simulink model "lazo_cerrado_cir"  (Simulink 7.6)
settings: Solver=VariableStepDiscrete  StartTime=0.0  StopTime=10.0  FixedStep=1e-3  MaxStep=1e-3  RelTol=1e0  AbsTol=1e1
values from neighbouring files (symbols this model uses):
  K = evalin('base','K')    [lazo_cerrado.m]    (also in linealizacion_dis.m = uquad_dlqr(Aext,Bext,Q,R); sim_lazo_cerrado.m = linealizacion_dis(modo,setpoint,0))
  setpoint = [evalin('base','vs') evalin('base','thetaps')]    [lazo_cerrado.m]    (also in programa_de_vuelo.m = [v(k,:) 0]; sim_lazo_cerrado.m = [ G(1) G(2) G(3) G(4) G(5) G(6) G(7) G(8)])
  thetap = evalin('base','thetap')    [linealizacion.m]
  ti = evalin('base','ti')    [lazo_cerrado.m]    (also in programa_de_vuelo.m = 0.1)
  Ts = evalin('base','Ts')    [linealizacion.m]    (also in linealizacion_dis.m)
undefined symbols (not defined in the file or in its folder): ang_amp, ang_frec, ang_offset, DiscIntNeverNeededParam, g, hor_amp, hor_frec, hor_offset, Ixx, Iyy, Izz, Izzm, L, M, phi0, psi0, theta0, vq10, vq20, vq30, vq_amp, vq_frec, vq_offset, wq10, wq20, wq30, wq_amp, wq_frec, wq_offset, x0, xc, y0, yaw_amp, yaw_frec, yaw_offset, yc, z0, z_amp, z_frec, z_offset, zc
libraries: commnoisgen2 x12, aerolibutil x3, simulink x1
settings Model: Creator=pater  LastModifiedBy=pater
settings SolverCC: InitialStep=0.01  MaxOrder=2  MaxConsecutiveMinStep=100  SolverJacobianMethodControl=FullPerturbation  SolverResetMethod=Robust
settings DataIOCC: SaveState=on
settings DebuggingCC: SignalInfNanChecking=error  MergeDetectMultiDrivingBlocksExec=warning

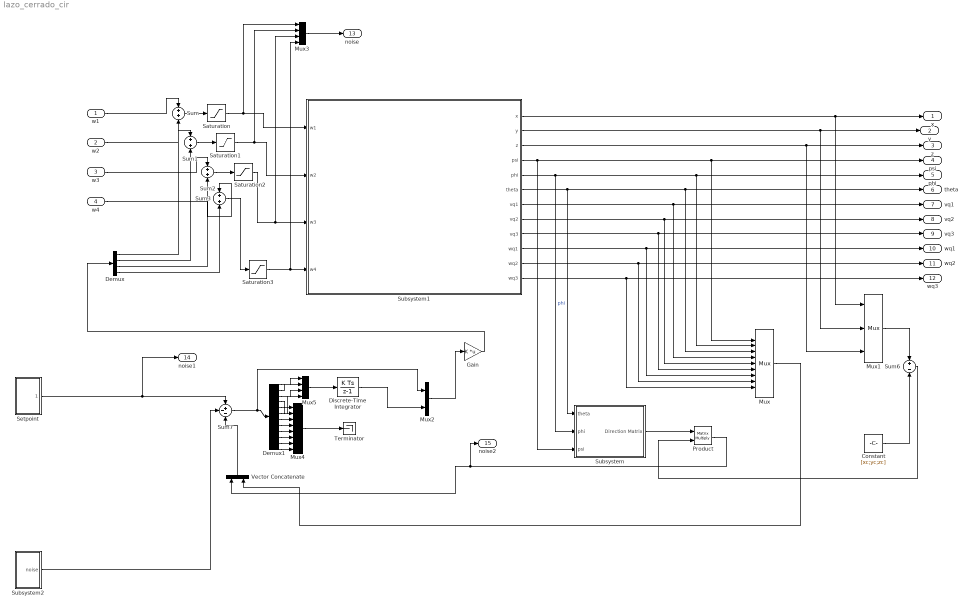
== system lazo_cerrado_cir ==
  w1 : Inport
  w2 : Inport  Port=2
  w3 : Inport  Port=3
  w4 : Inport  Port=4
  Constant : Constant  Value=[xc;yc;zc]
  Demux : Demux
  Demux1 : Demux  Outputs=12
  Discrete-Time Integrator : DiscreteIntegrator  SampleTime=Ts  UpperSaturationLimit=15  LowerSaturationLimit=-15  ICPrevOutput=DiscIntNeverNeededParam  ICPrevScaledInput=DiscIntNeverNeededParam
  Gain : Gain  Gain=K  Multiplication=Matrix(K*u) (u vector)
  Mux : Mux  Inputs=9
  Mux1 : Mux  Inputs=3
  Mux2 : Mux  Inputs=2
  Mux3 : Mux
  Mux4 : Mux  Inputs=8
  Mux5 : Mux
  Product : Product  Multiplication=Matrix(*)  RndMeth=Zero
  Saturation{,1..3} (4 alike) : Saturate  UpperLimit=387  LowerLimit=109
  Setpoint : Subsystem
  Subsystem : Subsystem
  Subsystem1 : Subsystem
  Subsystem2 : Subsystem
  Sum : Sum  OutMin=109.0  OutMax=387.0
  Sum1 : Sum  OutMin=109  OutMax=387
  Sum2 : Sum  OutMin=109  OutMax=387
  Sum3 : Sum  OutMin=109  OutMax=387
  Sum6 : Sum  Inputs=+-
  Sum7 : Sum  Inputs=+--
  Terminator : Terminator
  Vector Concatenate : Concatenate  Mode=Vector
  x : Outport
  y : Outport  Port=2
  z : Outport  Port=3  SampleTime=0.1
  psi : Outport  Port=4
  phi : Outport  Port=5
  theta : Outport  Port=6
  vq1 : Outport  Port=7
  vq2 : Outport  Port=8
  vq3 : Outport  Port=9
  wq1 : Outport  Port=10
  wq2 : Outport  Port=11
  wq3 : Outport  Port=12
  noise : Outport  Port=13
  noise1 : Outport  Port=14
  noise2 : Outport  Port=15
  wires:
  Subsystem1/1(x) -> x/1, Mux1/1
  Subsystem1/2(y) -> y/1, Mux1/2
  Subsystem1/3(z) -> z/1, Mux1/3
  Subsystem1/4(psi) -> psi/1, Mux/1, Subsystem/3(psi)
  Subsystem1/5(phi) -> Mux/2, phi/1, Subsystem/2(phi)  "phi"
  Subsystem1/6(theta) -> theta/1, Mux/3, Subsystem/1(theta)
  Subsystem1/7(vq1) -> vq1/1, Mux/4
  Subsystem1/8(vq2) -> vq2/1, Mux/5
  Subsystem1/9(vq3) -> vq3/1, Mux/6
  Subsystem1/10(wq1) -> wq1/1, Mux/7
  Subsystem1/11(wq2) -> wq2/1, Mux/8
  Subsystem1/12(wq3) -> wq3/1, Mux/9
  Mux/1 -> Vector Concatenate/2
  Mux1/1 -> Sum6/1
  Constant/1 -> Sum6/2
  Sum6/1 -> Product/2
  Subsystem/1(Direction Matrix) -> Product/1
  Demux/4 -> Sum3/2
  Demux/3 -> Sum2/2
  Demux/2 -> Sum1/2
  Demux/1 -> Sum/2
  w1/1 -> Sum/1
  w2/1 -> Sum1/1
  w3/1 -> Sum2/1
  w4/1 -> Sum3/1
  Sum3/1 -> Saturation3/1
  Sum2/1 -> Saturation2/1
  Sum1/1 -> Saturation1/1
  Sum/1 -> Saturation/1
  Saturation/1 -> Subsystem1/1(w1), Mux3/1
  Saturation1/1 -> Mux3/2, Subsystem1/2(w2)
  Saturation2/1 -> Subsystem1/3(w3), Mux3/3
  Saturation3/1 -> Subsystem1/4(w4), Mux3/4
  Gain/1 -> Demux/1
  Subsystem2/1(noise) -> Sum7/2
  Product/1 -> Vector Concatenate/1, noise2/1
  Sum7/1 -> Demux1/1, Mux2/1
  Mux4/1 -> Terminator/1
  Demux1/12 -> Mux4/8
  Demux1/11 -> Mux4/7
  Demux1/10 -> Mux4/6
  Demux1/9 -> Mux4/5
  Demux1/8 -> Mux4/4
  Demux1/7 -> Mux4/3
  Demux1/5 -> Mux4/2
  Demux1/4 -> Mux4/1
  Demux1/2 -> Mux5/2
  Demux1/1 -> Mux5/1
  Mux5/1 -> Discrete-Time Integrator/1
  Vector Concatenate/1 -> Sum7/3
  Setpoint/1(Setpoint) -> Sum7/1, noise1/1
  Mux3/1 -> noise/1
  Mux2/1 -> Gain/1
  Discrete-Time Integrator/1 -> Mux2/2
  Demux1/6 -> Mux5/4
  Demux1/3 -> Mux5/3

== system lazo_cerrado_cir/Setpoint ==
  Digital Clock : DigitalClock  SampleTime=Ts
  Product : Product  RndMeth=Zero
  Roll y Pitch : Constant  Value=[setpoint(4);setpoint(5)]
  Sum : Sum  Inputs=|++
  Sum1 : Sum  Inputs=|+-
  Vector Concatenate : Concatenate  NumInputs=4  Mode=Vector
  Vel y vel angular : Constant  Value=setpoint(6:11)
  Velocidad angular : Constant  Value=thetap
  angulo inicial : Constant  Value=theta0
  ti : Constant  Value=ti
  xq,yq,zq : Constant  Value=[setpoint(3);setpoint(2);setpoint(1)]
  Setpoint : Outport
  wires:
  Velocidad angular/1 -> Product/2
  Vector Concatenate/1 -> Setpoint/1
  angulo inicial/1 -> Sum/2
  ti/1 -> Sum1/2
  Digital Clock/1 -> Sum1/1
  Sum1/1 -> Product/1
  Product/1 -> Sum/1
  Vel y vel angular/1 -> Vector Concatenate/4
  Sum/1 -> Vector Concatenate/3
  Roll y Pitch/1 -> Vector Concatenate/2
  xq,yq,zq/1 -> Vector Concatenate/1

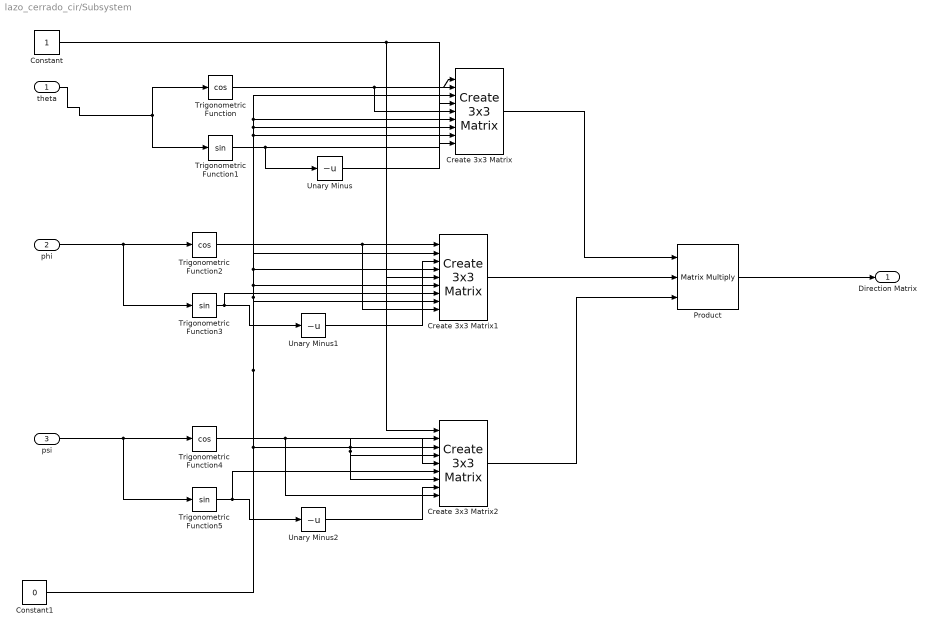
== system lazo_cerrado_cir/Subsystem ==
  theta : Inport
  phi : Inport  Port=2
  psi : Inport  Port=3
  Constant : Constant
  Constant1 : Constant  Value=0
  Create 3x3 Matrix : aerolibutil/Create 3x3 Matrix  SystemSampleTime=-1
  Create 3x3 Matrix1 : aerolibutil/Create 3x3 Matrix  SystemSampleTime=-1
  Create 3x3 Matrix2 : aerolibutil/Create 3x3 Matrix  SystemSampleTime=-1
  Product : Product  Inputs=3  Multiplication=Matrix(*)  RndMeth=Zero
  Trigonometric Function : Trigonometry  Operator=cos
  Trigonometric Function1 : Trigonometry
  Trigonometric Function2 : Trigonometry  Operator=cos
  Trigonometric Function3 : Trigonometry
  Trigonometric Function4 : Trigonometry  Operator=cos
  Trigonometric Function5 : Trigonometry
  Unary Minus : UnaryMinus
  Unary Minus1 : UnaryMinus
  Unary Minus2 : UnaryMinus
  Direction Matrix : Outport
  wires:
  Constant1/1 -> Create 3x3 Matrix/3, Create 3x3 Matrix/6, Create 3x3 Matrix/7, Create 3x3 Matrix/8, Create 3x3 Matrix1/2, Create 3x3 Matrix1/4, Create 3x3 Matrix1/6, Create 3x3 Matrix1/8, Create 3x3 Matrix2/3, Create 3x3 Matrix2/2, Create 3x3 Matrix2/7, Create 3x3 Matrix2/4
  Constant/1 -> Create 3x3 Matrix/9, Create 3x3 Matrix1/5, Create 3x3 Matrix2/1
  Trigonometric Function/1 -> Create 3x3 Matrix/1, Create 3x3 Matrix/5
  Trigonometric Function1/1 -> Create 3x3 Matrix/2, Unary Minus/1
  Unary Minus/1 -> Create 3x3 Matrix/4
  Trigonometric Function3/1 -> Unary Minus1/1, Create 3x3 Matrix1/7
  phi/1 -> Trigonometric Function2/1, Trigonometric Function3/1
  Trigonometric Function2/1 -> Create 3x3 Matrix1/1, Create 3x3 Matrix1/9
  Unary Minus1/1 -> Create 3x3 Matrix1/3
  Trigonometric Function5/1 -> Unary Minus2/1, Create 3x3 Matrix2/6
  psi/1 -> Trigonometric Function4/1, Trigonometric Function5/1
  Trigonometric Function4/1 -> Create 3x3 Matrix2/5, Create 3x3 Matrix2/9
  Unary Minus2/1 -> Create 3x3 Matrix2/8
  Product/1 -> Direction Matrix/1
  Create 3x3 Matrix1/1 -> Product/2
  Create 3x3 Matrix/1 -> Product/1
  Create 3x3 Matrix2/1 -> Product/3
  theta/1 -> Trigonometric Function/1, Trigonometric Function1/1

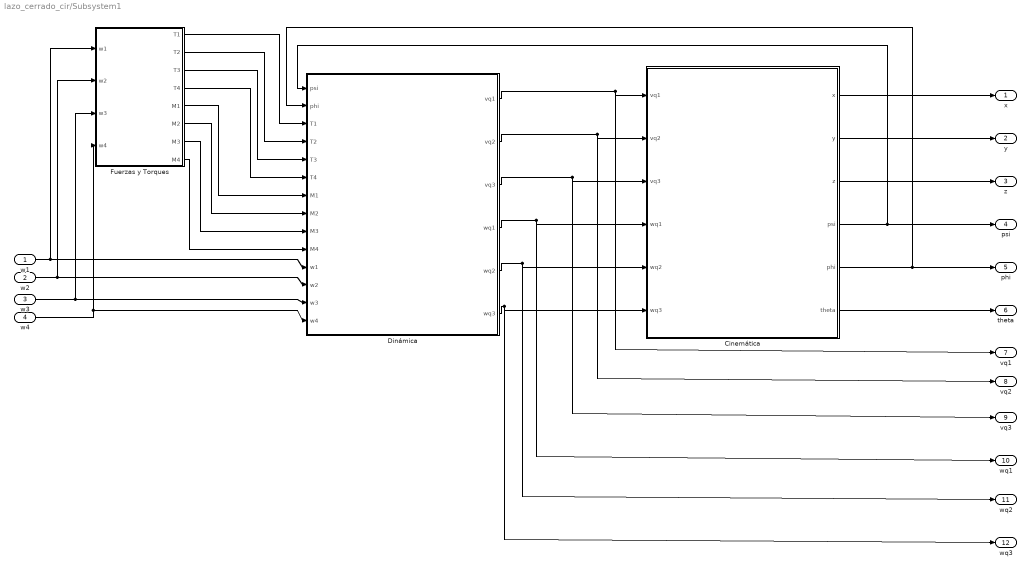
== system lazo_cerrado_cir/Subsystem1 ==
  w1 : Inport  OutMin=109  OutMax=387
  w2 : Inport  Port=2  OutMin=109  OutMax=387
  w3 : Inport  Port=3  OutMin=109  OutMax=387
  w4 : Inport  Port=4  OutMin=109  OutMax=387
  Cinemática : Subsystem
  Dinámica : Subsystem
  Fuerzas y Torques : Subsystem
  x : Outport
  y : Outport  Port=2
  z : Outport  Port=3
  psi : Outport  Port=4
  phi : Outport  Port=5
  theta : Outport  Port=6
  vq1 : Outport  Port=7
  vq2 : Outport  Port=8
  vq3 : Outport  Port=9
  wq1 : Outport  Port=10
  wq2 : Outport  Port=11
  wq3 : Outport  Port=12
  wires:
  Cinemática/1(x) -> x/1
  Cinemática/2(y) -> y/1
  Cinemática/3(z) -> z/1
  Cinemática/4(psi) -> psi/1, Dinámica/1(psi)
  Cinemática/5(phi) -> phi/1, Dinámica/2(phi)
  Cinemática/6(theta) -> theta/1
  w2/1 -> Fuerzas y Torques/2(w2), Dinámica/12(w2)
  w3/1 -> Fuerzas y Torques/3(w3), Dinámica/13(w3)
  w4/1 -> Fuerzas y Torques/4(w4), Dinámica/14(w4)
  Dinámica/6(wq3) -> wq3/1, Cinemática/6(wq3)
  Fuerzas y Torques/1(T1) -> Dinámica/3(T1)
  Fuerzas y Torques/2(T2) -> Dinámica/4(T2)
  Fuerzas y Torques/3(T3) -> Dinámica/5(T3)
  Fuerzas y Torques/4(T4) -> Dinámica/6(T4)
  Fuerzas y Torques/5(M1) -> Dinámica/7(M1)
  Fuerzas y Torques/6(M2) -> Dinámica/8(M2)
  Fuerzas y Torques/7(M3) -> Dinámica/9(M3)
  Fuerzas y Torques/8(M4) -> Dinámica/10(M4)
  w1/1 -> Fuerzas y Torques/1(w1), Dinámica/11(w1)
  Dinámica/1(vq1) -> Cinemática/1(vq1), vq1/1
  Dinámica/2(vq2) -> Cinemática/2(vq2), vq2/1
  Dinámica/3(vq3) -> Cinemática/3(vq3), vq3/1
  Dinámica/4(wq1) -> Cinemática/4(wq1), wq1/1
  Dinámica/5(wq2) -> Cinemática/5(wq2), wq2/1

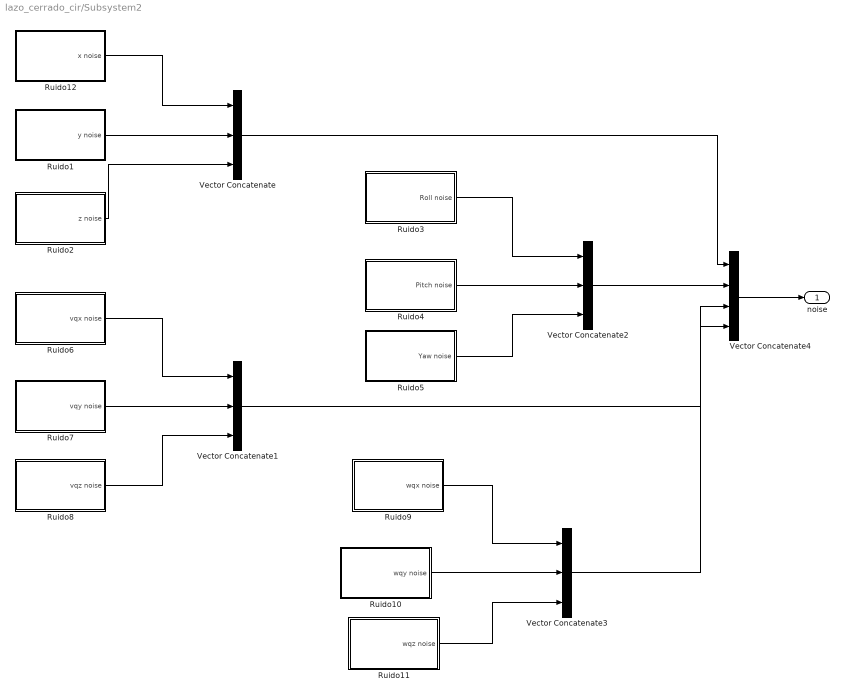
== system lazo_cerrado_cir/Subsystem2 ==
  Ruido1 : Subsystem
  Ruido10 : Subsystem
  Ruido11 : Subsystem
  Ruido12 : Subsystem
  Ruido2 : Subsystem
  Ruido3 : Subsystem
  Ruido4 : Subsystem
  Ruido5 : Subsystem
  Ruido6 : Subsystem
  Ruido7 : Subsystem
  Ruido8 : Subsystem
  Ruido9 : Subsystem
  Vector Concatenate{,1..3} (4 alike) : Concatenate  NumInputs=3  Mode=Vector
  Vector Concatenate4 : Concatenate  NumInputs=4  Mode=Vector
  noise : Outport
  wires:
  Ruido12/1(x noise) -> Vector Concatenate/1
  Ruido1/1(y noise) -> Vector Concatenate/2
  Ruido2/1(z noise) -> Vector Concatenate/3
  Ruido6/1(vqx noise) -> Vector Concatenate1/1
  Ruido7/1(vqy noise) -> Vector Concatenate1/2
  Ruido8/1(vqz noise) -> Vector Concatenate1/3
  Ruido3/1(Roll noise) -> Vector Concatenate2/1
  Ruido4/1(Pitch noise) -> Vector Concatenate2/2
  Ruido9/1(wqx noise) -> Vector Concatenate3/1
  Ruido10/1(wqy noise) -> Vector Concatenate3/2
  Ruido11/1(wqz noise) -> Vector Concatenate3/3
  Vector Concatenate/1 -> Vector Concatenate4/1
  Vector Concatenate2/1 -> Vector Concatenate4/2
  Vector Concatenate1/1 -> Vector Concatenate4/3
  Vector Concatenate3/1 -> Vector Concatenate4/4
  Vector Concatenate4/1 -> noise/1
  Ruido5/1(Yaw noise) -> Vector Concatenate2/3

== system lazo_cerrado_cir/Subsystem1/Cinemática ==
  vq1 : Inport
  vq2 : Inport  Port=2
  vq3 : Inport  Port=3
  wq1 : Inport  Port=4
  wq2 : Inport  Port=5
  wq3 : Inport  Port=6
  Posiciones : Subsystem
  Ángulos De Euler : Subsystem
  x : Outport
  y : Outport  Port=2
  z : Outport  Port=3
  psi : Outport  Port=4
  phi : Outport  Port=5
  theta : Outport  Port=6
  wires:
  Posiciones/1(x) -> x/1
  Posiciones/2(y) -> y/1
  Posiciones/3(z) -> z/1
  Ángulos De Euler/1(psi) -> psi/1, Posiciones/3(psi)
  Ángulos De Euler/2(phi) -> phi/1, Posiciones/2(phi)
  Ángulos De Euler/3(theta) -> theta/1, Posiciones/1(theta)
  vq1/1 -> Posiciones/4(vq1)
  vq2/1 -> Posiciones/5(vq2)
  vq3/1 -> Posiciones/6(vq3)
  wq1/1 -> Ángulos De Euler/1(wq1)
  wq2/1 -> Ángulos De Euler/2(wq2)
  wq3/1 -> Ángulos De Euler/3(wq3)

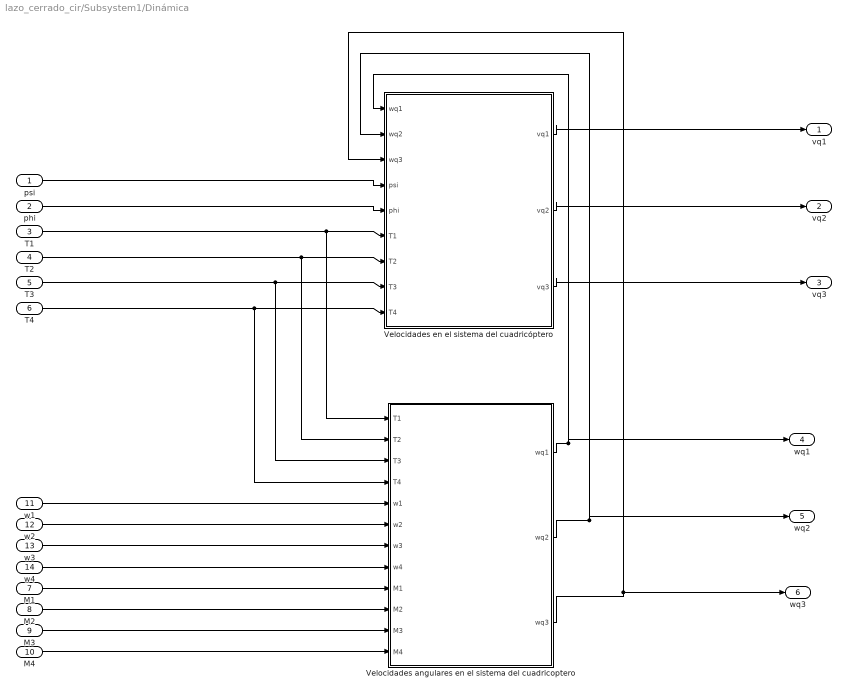
== system lazo_cerrado_cir/Subsystem1/Dinámica ==
  psi : Inport
  phi : Inport  Port=2
  T1 : Inport  Port=3
  T2 : Inport  Port=4
  T3 : Inport  Port=5
  T4 : Inport  Port=6
  M1 : Inport  Port=7
  M2 : Inport  Port=8
  M3 : Inport  Port=9
  M4 : Inport  Port=10
  w1 : Inport  Port=11
  w2 : Inport  Port=12
  w3 : Inport  Port=13
  w4 : Inport  Port=14
  Velocidades angulares en el sistema del cuadricoptero : Subsystem
  Velocidades en el sistema del cuadricóptero : Subsystem
  vq1 : Outport
  vq2 : Outport  Port=2
  vq3 : Outport  Port=3
  wq1 : Outport  Port=4
  wq2 : Outport  Port=5
  wq3 : Outport  Port=6
  wires:
  T1/1 -> Velocidades en el sistema del cuadricóptero/6(T1), Velocidades angulares en el sistema del cuadricoptero/1(T1)
  T2/1 -> Velocidades en el sistema del cuadricóptero/7(T2), Velocidades angulares en el sistema del cuadricoptero/2(T2)
  T3/1 -> Velocidades en el sistema del cuadricóptero/8(T3), Velocidades angulares en el sistema del cuadricoptero/3(T3)
  T4/1 -> Velocidades en el sistema del cuadricóptero/9(T4), Velocidades angulares en el sistema del cuadricoptero/4(T4)
  Velocidades angulares en el sistema del cuadricoptero/1(wq1) -> wq1/1, Velocidades en el sistema del cuadricóptero/1(wq1)
  Velocidades angulares en el sistema del cuadricoptero/2(wq2) -> wq2/1, Velocidades en el sistema del cuadricóptero/2(wq2)
  Velocidades angulares en el sistema del cuadricoptero/3(wq3) -> Velocidades en el sistema del cuadricóptero/3(wq3), wq3/1
  phi/1 -> Velocidades en el sistema del cuadricóptero/5(phi)
  psi/1 -> Velocidades en el sistema del cuadricóptero/4(psi)
  Velocidades en el sistema del cuadricóptero/3(vq3) -> vq3/1
  Velocidades en el sistema del cuadricóptero/2(vq2) -> vq2/1
  Velocidades en el sistema del cuadricóptero/1(vq1) -> vq1/1
  M2/1 -> Velocidades angulares en el sistema del cuadricoptero/10(M2)
  M3/1 -> Velocidades angulares en el sistema del cuadricoptero/11(M3)
  M4/1 -> Velocidades angulares en el sistema del cuadricoptero/12(M4)
  M1/1 -> Velocidades angulares en el sistema del cuadricoptero/9(M1)
  w1/1 -> Velocidades angulares en el sistema del cuadricoptero/5(w1)
  w2/1 -> Velocidades angulares en el sistema del cuadricoptero/6(w2)
  w3/1 -> Velocidades angulares en el sistema del cuadricoptero/7(w3)
  w4/1 -> Velocidades angulares en el sistema del cuadricoptero/8(w4)

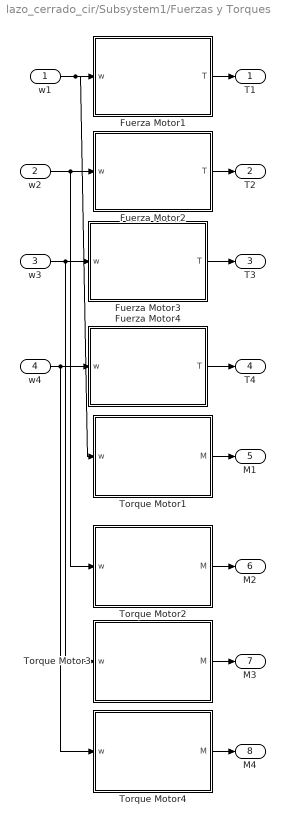
== system lazo_cerrado_cir/Subsystem1/Fuerzas y Torques ==
  w1 : Inport
  w2 : Inport  Port=2
  w3 : Inport  Port=3
  w4 : Inport  Port=4
  Fuerza Motor1 : Subsystem
  Fuerza Motor2 : Subsystem
  Fuerza Motor3 : Subsystem
  Fuerza Motor4 : Subsystem
  Torque Motor1 : Subsystem
  Torque Motor2 : Subsystem
  Torque Motor3 : Subsystem
  Torque Motor4 : Subsystem
  T1 : Outport
  T2 : Outport  Port=2
  T3 : Outport  Port=3
  T4 : Outport  Port=4
  M1 : Outport  Port=5
  M2 : Outport  Port=6
  M3 : Outport  Port=7
  M4 : Outport  Port=8
  wires:
  w1/1 -> Fuerza Motor1/1(w), Torque Motor1/1(w)
  w2/1 -> Torque Motor2/1(w), Fuerza Motor2/1(w)
  w3/1 -> Torque Motor3/1(w), Fuerza Motor3/1(w)
  w4/1 -> Torque Motor4/1(w), Fuerza Motor4/1(w)
  Fuerza Motor1/1(T) -> T1/1
  Fuerza Motor2/1(T) -> T2/1
  Fuerza Motor3/1(T) -> T3/1
  Fuerza Motor4/1(T) -> T4/1
  Torque Motor1/1(M) -> M1/1
  Torque Motor2/1(M) -> M2/1
  Torque Motor3/1(M) -> M3/1
  Torque Motor4/1(M) -> M4/1

== system lazo_cerrado_cir/Subsystem2/Ruido1 ==
  Add : Sum
  Digital Clock : DigitalClock
  Gain2 : Gain  Gain=2*pi*hor_frec
  Gain3 : Gain  Gain=hor_amp
  Gaussian Noise Generator : commnoisgen2/Gaussian Noise Generator  SystemSampleTime=-1  m=hor_offset  d=hor_cov  s=41  Ts=1  frameBased=off  sampPerFrame=1  orient=off  outDataType=double
  Trigonometric Function1 : Trigonometry
  y noise : Outport
  wires:
  Digital Clock/1 -> Gain2/1
  Gain2/1 -> Trigonometric Function1/1
  Trigonometric Function1/1 -> Gain3/1
  Add/1 -> y noise/1
  Gain3/1 -> Add/1
  Gaussian Noise Generator/1 -> Add/2

== system lazo_cerrado_cir/Subsystem2/Ruido10 ==
  Add : Sum
  Digital Clock : DigitalClock  SampleTime=Ts
  Gain2 : Gain  Gain=2*pi*wq_frec
  Gain3 : Gain  Gain=wq_amp
  Gaussian Noise Generator : commnoisgen2/Gaussian Noise Generator  SystemSampleTime=-1  m=wq_offset  d=wq_cov  s=41  Ts=Ts  frameBased=off  sampPerFrame=1  orient=off  outDataType=double
  Trigonometric Function1 : Trigonometry
  wqy noise : Outport
  wires:
  Digital Clock/1 -> Gain2/1
  Gain2/1 -> Trigonometric Function1/1
  Trigonometric Function1/1 -> Gain3/1
  Add/1 -> wqy noise/1
  Gain3/1 -> Add/1
  Gaussian Noise Generator/1 -> Add/2

== system lazo_cerrado_cir/Subsystem2/Ruido11 ==
  Add : Sum
  Digital Clock : DigitalClock  SampleTime=Ts
  Gain2 : Gain  Gain=2*pi*wq_frec
  Gain3 : Gain  Gain=wq_amp
  Gaussian Noise Generator : commnoisgen2/Gaussian Noise Generator  SystemSampleTime=-1  m=wq_offset  d=wq_cov  s=41  Ts=Ts  frameBased=off  sampPerFrame=1  orient=off  outDataType=double
  Trigonometric Function1 : Trigonometry
  wqz noise : Outport
  wires:
  Digital Clock/1 -> Gain2/1
  Gain2/1 -> Trigonometric Function1/1
  Trigonometric Function1/1 -> Gain3/1
  Add/1 -> wqz noise/1
  Gain3/1 -> Add/1
  Gaussian Noise Generator/1 -> Add/2

== system lazo_cerrado_cir/Subsystem2/Ruido12 ==
  Add : Sum
  Digital Clock : DigitalClock
  Gain2 : Gain  Gain=2*pi*hor_frec
  Gain3 : Gain  Gain=hor_amp
  Gaussian Noise Generator : commnoisgen2/Gaussian Noise Generator  SystemSampleTime=-1  m=hor_offset  d=hor_cov  s=41  Ts=1  frameBased=off  sampPerFrame=1  orient=off  outDataType=double
  Trigonometric Function1 : Trigonometry
  x noise : Outport
  wires:
  Digital Clock/1 -> Gain2/1
  Gain2/1 -> Trigonometric Function1/1
  Trigonometric Function1/1 -> Gain3/1
  Add/1 -> x noise/1
  Gain3/1 -> Add/1
  Gaussian Noise Generator/1 -> Add/2

== system lazo_cerrado_cir/Subsystem2/Ruido2 ==
  Add : Sum
  Digital Clock : DigitalClock  SampleTime=Ts
  Gain2 : Gain  Gain=2*pi*z_frec
  Gain3 : Gain  Gain=z_amp
  Gaussian Noise Generator : commnoisgen2/Gaussian Noise Generator  SystemSampleTime=-1  m=z_offset  d=z_cov  s=41  Ts=Ts  frameBased=off  sampPerFrame=1  orient=off  outDataType=double
  Trigonometric Function1 : Trigonometry
  z noise : Outport
  wires:
  Digital Clock/1 -> Gain2/1
  Gain2/1 -> Trigonometric Function1/1
  Trigonometric Function1/1 -> Gain3/1
  Add/1 -> z noise/1
  Gain3/1 -> Add/1
  Gaussian Noise Generator/1 -> Add/2

== system lazo_cerrado_cir/Subsystem2/Ruido3 ==
  Add : Sum
  Digital Clock : DigitalClock  SampleTime=Ts
  Gain2 : Gain  Gain=2*pi*ang_frec
  Gain3 : Gain  Gain=ang_amp
  Gaussian Noise Generator : commnoisgen2/Gaussian Noise Generator  SystemSampleTime=-1  m=ang_offset  d=ang_cov  s=41  Ts=Ts  frameBased=off  sampPerFrame=1  orient=off  outDataType=double
  Trigonometric Function1 : Trigonometry
  Roll noise : Outport
  wires:
  Digital Clock/1 -> Gain2/1
  Gain2/1 -> Trigonometric Function1/1
  Trigonometric Function1/1 -> Gain3/1
  Add/1 -> Roll noise/1
  Gain3/1 -> Add/1
  Gaussian Noise Generator/1 -> Add/2

== system lazo_cerrado_cir/Subsystem2/Ruido4 ==
  Add : Sum
  Digital Clock : DigitalClock  SampleTime=Ts
  Gain2 : Gain  Gain=2*pi*ang_frec
  Gain3 : Gain  Gain=ang_amp
  Gaussian Noise Generator : commnoisgen2/Gaussian Noise Generator  SystemSampleTime=-1  m=ang_offset  d=ang_cov  s=41  Ts=Ts  frameBased=off  sampPerFrame=1  orient=off  outDataType=double
  Trigonometric Function1 : Trigonometry
  Pitch noise : Outport
  wires:
  Digital Clock/1 -> Gain2/1
  Gain2/1 -> Trigonometric Function1/1
  Trigonometric Function1/1 -> Gain3/1
  Add/1 -> Pitch noise/1
  Gain3/1 -> Add/1
  Gaussian Noise Generator/1 -> Add/2

== system lazo_cerrado_cir/Subsystem2/Ruido5 ==
  Add : Sum
  Digital Clock : DigitalClock  SampleTime=Ts
  Gain2 : Gain  Gain=2*pi*yaw_frec
  Gain3 : Gain  Gain=yaw_amp
  Gaussian Noise Generator : commnoisgen2/Gaussian Noise Generator  SystemSampleTime=-1  m=yaw_offset  d=yaw_cov  s=41  Ts=Ts  frameBased=off  sampPerFrame=1  orient=off  outDataType=double
  Trigonometric Function1 : Trigonometry
  Yaw noise : Outport
  wires:
  Digital Clock/1 -> Gain2/1
  Gain2/1 -> Trigonometric Function1/1
  Trigonometric Function1/1 -> Gain3/1
  Add/1 -> Yaw noise/1
  Gain3/1 -> Add/1
  Gaussian Noise Generator/1 -> Add/2

== system lazo_cerrado_cir/Subsystem2/Ruido6 ==
  Add : Sum
  Digital Clock : DigitalClock  SampleTime=Ts
  Gain2 : Gain  Gain=2*pi*vq_frec
  Gain3 : Gain  Gain=vq_amp
  Gaussian Noise Generator : commnoisgen2/Gaussian Noise Generator  SystemSampleTime=-1  m=vq_offset  d=vq_cov  s=41  Ts=Ts  frameBased=off  sampPerFrame=1  orient=off  outDataType=double
  Trigonometric Function1 : Trigonometry
  vqx noise : Outport
  wires:
  Digital Clock/1 -> Gain2/1
  Gain2/1 -> Trigonometric Function1/1
  Trigonometric Function1/1 -> Gain3/1
  Add/1 -> vqx noise/1
  Gain3/1 -> Add/1
  Gaussian Noise Generator/1 -> Add/2

== system lazo_cerrado_cir/Subsystem2/Ruido7 ==
  Add : Sum
  Digital Clock : DigitalClock  SampleTime=Ts
  Gain2 : Gain  Gain=2*pi*vq_frec
  Gain3 : Gain  Gain=vq_amp
  Gaussian Noise Generator : commnoisgen2/Gaussian Noise Generator  SystemSampleTime=-1  m=vq_offset  d=vq_cov  s=41  Ts=Ts  frameBased=off  sampPerFrame=1  orient=off  outDataType=double
  Trigonometric Function1 : Trigonometry
  vqy noise : Outport
  wires:
  Digital Clock/1 -> Gain2/1
  Gain2/1 -> Trigonometric Function1/1
  Trigonometric Function1/1 -> Gain3/1
  Add/1 -> vqy noise/1
  Gain3/1 -> Add/1
  Gaussian Noise Generator/1 -> Add/2

== system lazo_cerrado_cir/Subsystem2/Ruido8 ==
  Add : Sum
  Digital Clock : DigitalClock  SampleTime=Ts
  Gain2 : Gain  Gain=2*pi*vq_frec
  Gain3 : Gain  Gain=vq_amp
  Gaussian Noise Generator : commnoisgen2/Gaussian Noise Generator  SystemSampleTime=-1  m=vq_offset  d=vq_cov  s=41  Ts=Ts  frameBased=off  sampPerFrame=1  orient=off  outDataType=double
  Trigonometric Function1 : Trigonometry
  vqz noise : Outport
  wires:
  Digital Clock/1 -> Gain2/1
  Gain2/1 -> Trigonometric Function1/1
  Trigonometric Function1/1 -> Gain3/1
  Add/1 -> vqz noise/1
  Gain3/1 -> Add/1
  Gaussian Noise Generator/1 -> Add/2

== system lazo_cerrado_cir/Subsystem2/Ruido9 ==
  Add : Sum
  Digital Clock : DigitalClock  SampleTime=Ts
  Gain2 : Gain  Gain=2*pi*wq_frec
  Gain3 : Gain  Gain=wq_amp
  Gaussian Noise Generator : commnoisgen2/Gaussian Noise Generator  SystemSampleTime=-1  m=wq_offset  d=wq_cov  s=41  Ts=Ts  frameBased=off  sampPerFrame=1  orient=off  outDataType=double
  Trigonometric Function1 : Trigonometry
  wqx noise : Outport
  wires:
  Digital Clock/1 -> Gain2/1
  Gain2/1 -> Trigonometric Function1/1
  Trigonometric Function1/1 -> Gain3/1
  Add/1 -> wqx noise/1
  Gain3/1 -> Add/1
  Gaussian Noise Generator/1 -> Add/2

== system lazo_cerrado_cir/Subsystem1/Cinemática/Posiciones ==
  theta : Inport
  phi : Inport  Port=2
  psi : Inport  Port=3
  vq1 : Inport  Port=4
  vq2 : Inport  Port=5
  vq3 : Inport  Port=6
  Subsystem3 : Subsystem
  Subsystem4 : Subsystem
  Subsystem5 : Subsystem
  x : Outport
  y : Outport  Port=2
  z : Outport  Port=3
  wires:
  Subsystem3/1(x) -> x/1
  Subsystem4/1(y) -> y/1
  Subsystem5/1(z) -> z/1
  vq3/1 -> Subsystem5/5(vq3), Subsystem4/6(vq3), Subsystem3/6(vq3)
  theta/1 -> Subsystem3/1(theta), Subsystem4/1(theta)
  phi/1 -> Subsystem3/2(phi), Subsystem4/2(phi), Subsystem5/1(phi)
  psi/1 -> Subsystem3/3(psi), Subsystem4/3(psi), Subsystem5/2(psi)
  vq2/1 -> Subsystem5/4(vq2), Subsystem4/5(vq2), Subsystem3/5(vq2)
  vq1/1 -> Subsystem5/3(vq1), Subsystem4/4(vq1), Subsystem3/4(vq1)

== system lazo_cerrado_cir/Subsystem1/Cinemática/Ángulos De Euler ==
  wq1 : Inport
  wq2 : Inport  Port=2
  wq3 : Inport  Port=3
  Subsystem : Subsystem
  Subsystem1 : Subsystem
  Subsystem2 : Subsystem
  psi : Outport
  phi : Outport  Port=2
  theta : Outport  Port=3
  wires:
  Subsystem1/1(psi) -> psi/1, Subsystem/1(psi), Subsystem2/1(psi)
  Subsystem2/1(phi) -> phi/1, Subsystem/2(phi), Subsystem1/1(phi)
  Subsystem/1(theta) -> theta/1
  wq3/1 -> Subsystem/4(wq3), Subsystem2/3(wq3), Subsystem1/2(wq3)
  wq1/1 -> Subsystem1/4(wq1)
  wq2/1 -> Subsystem2/2(wq2), Subsystem1/3(wq2), Subsystem/3(wq2)

== system lazo_cerrado_cir/Subsystem1/Dinámica/Velocidades angulares en el sistema del cuadricoptero ==
  T1 : Inport
  T2 : Inport  Port=2
  T3 : Inport  Port=3
  T4 : Inport  Port=4
  w1 : Inport  Port=5
  w2 : Inport  Port=6
  w3 : Inport  Port=7
  w4 : Inport  Port=8
  M1 : Inport  Port=9
  M2 : Inport  Port=10
  M3 : Inport  Port=11
  M4 : Inport  Port=12
  Subsystem10 : Subsystem
  Subsystem11 : Subsystem
  Subsystem9 : Subsystem
  wq1 : Outport
  wq2 : Outport  Port=2
  wq3 : Outport  Port=3
  wires:
  Subsystem9/1(wq1) -> wq1/1, Subsystem11/1(wq1), Subsystem10/1(wq1)
  Subsystem10/1(wq2) -> wq2/1, Subsystem11/2(wq2), Subsystem9/1(wq2)
  Subsystem11/1(wq3) -> wq3/1, Subsystem10/2(wq3), Subsystem9/2(wq3)
  w4/1 -> Subsystem11/6(w4), Subsystem10/8(w4), Subsystem9/8(w4)
  w3/1 -> Subsystem11/5(w3), Subsystem10/7(w3), Subsystem9/7(w3)
  w2/1 -> Subsystem11/4(w2), Subsystem10/6(w2), Subsystem9/6(w2)
  w1/1 -> Subsystem11/3(w1), Subsystem10/5(w1), Subsystem9/5(w1)
  T3/1 -> Subsystem10/4(T3)
  T1/1 -> Subsystem10/3(T1)
  T2/1 -> Subsystem9/4(T2)
  T4/1 -> Subsystem9/3(T4)
  M1/1 -> Subsystem11/7(M1)
  M2/1 -> Subsystem11/8(M2)
  M3/1 -> Subsystem11/9(M3)
  M4/1 -> Subsystem11/10(M4)

== system lazo_cerrado_cir/Subsystem1/Dinámica/Velocidades en el sistema del cuadricóptero ==
  wq1 : Inport
  wq2 : Inport  Port=2
  wq3 : Inport  Port=3
  psi : Inport  Port=4
  phi : Inport  Port=5
  T1 : Inport  Port=6
  T2 : Inport  Port=7
  T3 : Inport  Port=8
  T4 : Inport  Port=9
  Subsystem6 : Subsystem
  Subsystem7 : Subsystem
  Subsystem8 : Subsystem
  vq1 : Outport
  vq2 : Outport  Port=2
  vq3 : Outport  Port=3
  wires:
  Subsystem6/1(vq1) -> vq1/1, Subsystem8/5(vq1), Subsystem7/7(vq1), Subsystem7/8(vq2)
  Subsystem8/1(vq2) -> Subsystem6/4(vq2), vq2/1
  Subsystem7/1(vq3) -> vq3/1, Subsystem6/5(vq3), Subsystem8/4(vq3)
  wq1/1 -> Subsystem8/3(wq1), Subsystem7/1(wq1)
  wq3/1 -> Subsystem6/3(wq3), Subsystem8/2(wq3)
  psi/1 -> Subsystem8/6(psi), Subsystem7/10(psi)
  phi/1 -> Subsystem6/1(phi), Subsystem8/1(phi), Subsystem7/9(phi)
  wq2/1 -> Subsystem6/2(wq2), Subsystem7/2(wq2)
  T1/1 -> Subsystem7/3(T1)
  T2/1 -> Subsystem7/4(T2)
  T3/1 -> Subsystem7/5(T3)
  T4/1 -> Subsystem7/6(T4)

== system lazo_cerrado_cir/Subsystem1/Fuerzas y Torques/Fuerza Motor1 ==
  w : Inport
  Add : Sum
  Gain : Gain  Gain=4.60160135072435e-05
  Gain1 : Gain  Gain=-0.001038227262737266741675
  Product : Product  RndMeth=Zero
  T : Outport
  wires:
  Add/1 -> T/1
  Gain1/1 -> Add/2
  Product/1 -> Gain/1
  Gain/1 -> Add/1
  w/1 -> Gain1/1, Product/2, Product/1

== system lazo_cerrado_cir/Subsystem1/Fuerzas y Torques/Fuerza Motor2 ==
  w : Inport
  Add : Sum
  Gain : Gain  Gain=4.60160135072435e-05
  Gain1 : Gain  Gain=-0.001038227262737266741675
  Product : Product  RndMeth=Zero
  T : Outport
  wires:
  Add/1 -> T/1
  Gain1/1 -> Add/2
  Product/1 -> Gain/1
  Gain/1 -> Add/1
  w/1 -> Gain1/1, Product/2, Product/1

== system lazo_cerrado_cir/Subsystem1/Fuerzas y Torques/Fuerza Motor3 ==
  w : Inport
  Add : Sum
  Gain : Gain  Gain=4.60160135072435e-05
  Gain1 : Gain  Gain=-0.001038227262737266741675
  Product : Product  RndMeth=Zero
  T : Outport
  wires:
  Add/1 -> T/1
  Gain1/1 -> Add/2
  Product/1 -> Gain/1
  Gain/1 -> Add/1
  w/1 -> Gain1/1, Product/2, Product/1

== system lazo_cerrado_cir/Subsystem1/Fuerzas y Torques/Fuerza Motor4 ==
  w : Inport
  Add : Sum
  Gain : Gain  Gain=4.60160135072435e-05
  Gain1 : Gain  Gain=-0.001038227262737266741675
  Product : Product  RndMeth=Zero
  T : Outport
  wires:
  Add/1 -> T/1
  Gain1/1 -> Add/2
  Product/1 -> Gain/1
  Gain/1 -> Add/1
  w/1 -> Gain1/1, Product/2, Product/1

== system lazo_cerrado_cir/Subsystem1/Fuerzas y Torques/Torque Motor1 ==
  w : Inport
  Add : Sum
  Gain : Gain  Gain=3.4734e-6
  Gain1 : Gain  Gain=-1.3205e-4
  Product : Product  RndMeth=Zero
  M : Outport
  wires:
  Add/1 -> M/1
  Gain1/1 -> Add/2
  Product/1 -> Gain/1
  Gain/1 -> Add/1
  w/1 -> Gain1/1, Product/2, Product/1

== system lazo_cerrado_cir/Subsystem1/Fuerzas y Torques/Torque Motor2 ==
  w : Inport
  Add : Sum
  Gain : Gain  Gain=3.4734e-6
  Gain1 : Gain  Gain=-1.3205e-4
  Product : Product  RndMeth=Zero
  M : Outport
  wires:
  Add/1 -> M/1
  Gain1/1 -> Add/2
  Product/1 -> Gain/1
  Gain/1 -> Add/1
  w/1 -> Gain1/1, Product/2, Product/1

== system lazo_cerrado_cir/Subsystem1/Fuerzas y Torques/Torque Motor3 ==
  w : Inport
  Add : Sum
  Gain : Gain  Gain=3.4734e-6
  Gain1 : Gain  Gain=-1.3205e-4
  Product : Product  RndMeth=Zero
  M : Outport
  wires:
  Add/1 -> M/1
  Gain1/1 -> Add/2
  Product/1 -> Gain/1
  Gain/1 -> Add/1
  w/1 -> Gain1/1, Product/2, Product/1

== system lazo_cerrado_cir/Subsystem1/Fuerzas y Torques/Torque Motor4 ==
  w : Inport
  Add : Sum
  Gain : Gain  Gain=3.4734e-6
  Gain1 : Gain  Gain=-1.3205e-4
  Product : Product  RndMeth=Zero
  M : Outport
  wires:
  Add/1 -> M/1
  Gain1/1 -> Add/2
  Product/1 -> Gain/1
  Gain/1 -> Add/1
  w/1 -> Gain1/1, Product/2, Product/1

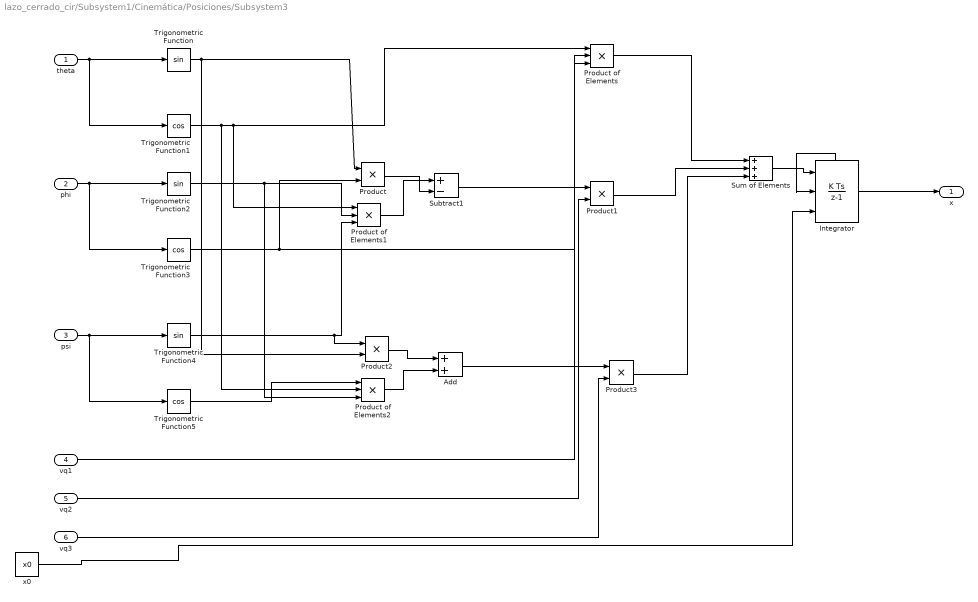
== system lazo_cerrado_cir/Subsystem1/Cinemática/Posiciones/Subsystem3 ==
  theta : Inport
  phi : Inport  Port=2
  psi : Inport  Port=3
  vq1 : Inport  Port=4
  vq2 : Inport  Port=5
  vq3 : Inport  Port=6
  Add : Sum
  Integrator : DiscreteIntegrator  ExternalReset=either  InitialConditionSource=external  SampleTime=Ts  ShowStatePort=on  ICPrevOutput=DiscIntNeverNeededParam  ICPrevScaledInput=DiscIntNeverNeededParam  mask(DiscretizedDiscreteIntegrator){}
      mask init:
      | %zoh
  Product{,1..3} (4 alike) : Product  RndMeth=Zero
  Product of Elements : Product  Inputs=3
  Product of Elements1 : Product  Inputs=3
  Product of Elements2 : Product  Inputs=3
  Subtract1 : Sum  Inputs=+-
  Sum of Elements : Sum  Inputs=3
  Trigonometric Function : Trigonometry
  Trigonometric Function1 : Trigonometry  Operator=cos
  Trigonometric Function2 : Trigonometry
  Trigonometric Function3 : Trigonometry  Operator=cos
  Trigonometric Function4 : Trigonometry
  Trigonometric Function5 : Trigonometry  Operator=cos
  x0 : Constant  Value=x0
  x : Outport
  wires:
  theta/1 -> Trigonometric Function/1, Trigonometric Function1/1
  phi/1 -> Trigonometric Function2/1, Trigonometric Function3/1
  psi/1 -> Trigonometric Function4/1, Trigonometric Function5/1
  Trigonometric Function1/1 -> Product of Elements/1, Product of Elements1/1, Product of Elements2/2
  Trigonometric Function3/1 -> Product of Elements/2, Product/2
  vq1/1 -> Product of Elements/3
  Trigonometric Function/1 -> Product/1, Product2/2
  Trigonometric Function2/1 -> Product of Elements1/2, Product of Elements2/3
  Trigonometric Function4/1 -> Product of Elements1/3, Product2/1
  Subtract1/1 -> Product1/1
  vq2/1 -> Product1/2
  Product2/1 -> Add/1
  Product of Elements2/1 -> Add/2
  Trigonometric Function5/1 -> Product of Elements2/1
  Add/1 -> Product3/1
  vq3/1 -> Product3/2
  Product of Elements/1 -> Sum of Elements/1
  Product1/1 -> Sum of Elements/2
  Product3/1 -> Sum of Elements/3
  Sum of Elements/1 -> Integrator/1
  Integrator/1 -> x/1
  Product of Elements1/1 -> Subtract1/1
  Product/1 -> Subtract1/2
  x0/1 -> Integrator/3
  Integrator/State -> Integrator/2

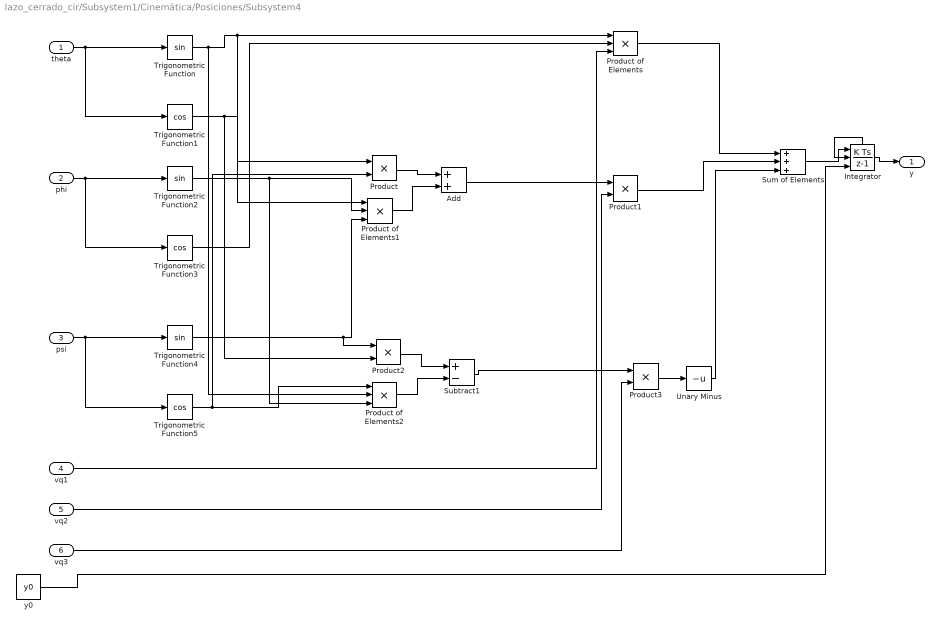
== system lazo_cerrado_cir/Subsystem1/Cinemática/Posiciones/Subsystem4 ==
  theta : Inport
  phi : Inport  Port=2
  psi : Inport  Port=3
  vq1 : Inport  Port=4
  vq2 : Inport  Port=5
  vq3 : Inport  Port=6
  Add : Sum
  Integrator : DiscreteIntegrator  ExternalReset=either  InitialConditionSource=external  SampleTime=Ts  ShowStatePort=on  ICPrevOutput=DiscIntNeverNeededParam  ICPrevScaledInput=DiscIntNeverNeededParam  mask(DiscretizedDiscreteIntegrator){}
      mask init:
      | %zoh
  Product{,1..3} (4 alike) : Product  RndMeth=Zero
  Product of Elements : Product  Inputs=3
  Product of Elements1 : Product  Inputs=3
  Product of Elements2 : Product  Inputs=3
  Subtract1 : Sum  Inputs=+-
  Sum of Elements : Sum  Inputs=3
  Trigonometric Function : Trigonometry
  Trigonometric Function1 : Trigonometry  Operator=cos
  Trigonometric Function2 : Trigonometry
  Trigonometric Function3 : Trigonometry  Operator=cos
  Trigonometric Function4 : Trigonometry
  Trigonometric Function5 : Trigonometry  Operator=cos
  Unary Minus : UnaryMinus
  y0 : Constant  Value=y0
  y : Outport
  wires:
  theta/1 -> Trigonometric Function/1, Trigonometric Function1/1
  phi/1 -> Trigonometric Function2/1, Trigonometric Function3/1
  psi/1 -> Trigonometric Function4/1, Trigonometric Function5/1
  Trigonometric Function1/1 -> Product/1, Product2/2
  Trigonometric Function3/1 -> Product of Elements/2
  vq1/1 -> Product of Elements/3
  Trigonometric Function/1 -> Product of Elements/1, Product of Elements1/1, Product of Elements2/2
  Trigonometric Function2/1 -> Product of Elements1/2, Product of Elements2/3
  Trigonometric Function4/1 -> Product of Elements1/3, Product2/1
  Product/1 -> Add/1
  Product of Elements1/1 -> Add/2
  Add/1 -> Product1/1
  vq2/1 -> Product1/2
  Trigonometric Function5/1 -> Product of Elements2/1, Product/2
  Subtract1/1 -> Product3/1
  vq3/1 -> Product3/2
  Product of Elements/1 -> Sum of Elements/1
  Product1/1 -> Sum of Elements/2
  Product3/1 -> Unary Minus/1
  Sum of Elements/1 -> Integrator/1
  Integrator/1 -> y/1
  Unary Minus/1 -> Sum of Elements/3
  Product of Elements2/1 -> Subtract1/2
  Product2/1 -> Subtract1/1
  y0/1 -> Integrator/3
  Integrator/State -> Integrator/2

== system lazo_cerrado_cir/Subsystem1/Cinemática/Posiciones/Subsystem5 ==
  phi : Inport
  psi : Inport  Port=2
  vq1 : Inport  Port=3
  vq2 : Inport  Port=4
  vq3 : Inport  Port=5
  Integrator : DiscreteIntegrator  ExternalReset=either  InitialConditionSource=external  SampleTime=Ts  ShowStatePort=on  ICPrevOutput=DiscIntNeverNeededParam  ICPrevScaledInput=DiscIntNeverNeededParam  mask(DiscretizedDiscreteIntegrator){}
      mask init:
      | %zoh
  Product : Product  RndMeth=Zero
  Product of Elements : Product  Inputs=3
  Product of Elements1 : Product  Inputs=3
  Sum of Elements : Sum  Inputs=3
  Trigonometric Function2 : Trigonometry
  Trigonometric Function3 : Trigonometry  Operator=cos
  Trigonometric Function4 : Trigonometry
  Trigonometric Function5 : Trigonometry  Operator=cos
  Unary Minus : UnaryMinus
  z0 : Constant  Value=z0
  z : Outport
  wires:
  phi/1 -> Trigonometric Function2/1, Trigonometric Function3/1
  psi/1 -> Trigonometric Function4/1, Trigonometric Function5/1
  Sum of Elements/1 -> Integrator/1
  Integrator/1 -> z/1
  Trigonometric Function2/1 -> Product/1
  vq1/1 -> Product/2
  Product/1 -> Unary Minus/1
  Trigonometric Function3/1 -> Product of Elements/1, Product of Elements1/1
  Trigonometric Function4/1 -> Product of Elements/2
  vq2/1 -> Product of Elements/3
  Trigonometric Function5/1 -> Product of Elements1/2
  vq3/1 -> Product of Elements1/3
  Product of Elements/1 -> Sum of Elements/2
  Product of Elements1/1 -> Sum of Elements/3
  Unary Minus/1 -> Sum of Elements/1
  z0/1 -> Integrator/3
  Integrator/State -> Integrator/2

== system lazo_cerrado_cir/Subsystem1/Cinemática/Ángulos De Euler/Subsystem ==
  psi : Inport
  phi : Inport  Port=2
  wq2 : Inport  Port=3
  wq3 : Inport  Port=4
  Divide : Product  Inputs=*/
  Integrator : DiscreteIntegrator  InitialConditionSource=external  SampleTime=Ts  ICPrevOutput=DiscIntNeverNeededParam  ICPrevScaledInput=DiscIntNeverNeededParam  mask(DiscretizedDiscreteIntegrator){}
      mask init:
      | %zoh
  Product : Product  RndMeth=Zero
  Product1 : Product  RndMeth=Zero
  Sum : Sum  Inputs=|++
  Trigonometric Function : Trigonometry  Operator=cos
  Trigonometric Function1 : Trigonometry
  Trigonometric Function2 : Trigonometry  Operator=cos
  theta0 : Constant  Value=theta0
  theta : Outport
  wires:
  wq3/1 -> Product/1
  wq2/1 -> Product1/1
  Product/1 -> Sum/1
  Product1/1 -> Sum/2
  Sum/1 -> Divide/1
  Trigonometric Function2/1 -> Divide/2
  Divide/1 -> Integrator/1
  Trigonometric Function/1 -> Product/2
  Trigonometric Function1/1 -> Product1/2
  phi/1 -> Trigonometric Function2/1
  Integrator/1 -> theta/1
  psi/1 -> Trigonometric Function/1, Trigonometric Function1/1
  theta0/1 -> Integrator/2

== system lazo_cerrado_cir/Subsystem1/Cinemática/Ángulos De Euler/Subsystem1 ==
  phi : Inport
  wq3 : Inport  Port=2
  wq2 : Inport  Port=3
  wq1 : Inport  Port=4
  Add : Sum
  Integrator : DiscreteIntegrator  InitialConditionSource=external  SampleTime=Ts  ICPrevOutput=DiscIntNeverNeededParam  ICPrevScaledInput=DiscIntNeverNeededParam  mask(DiscretizedDiscreteIntegrator){}
      mask init:
      | %zoh
  Product : Product  RndMeth=Zero
  Product1 : Product  RndMeth=Zero
  Product2 : Product  RndMeth=Zero
  Sum : Sum  Inputs=|++
  Trigonometric Function : Trigonometry
  Trigonometric Function2 : Trigonometry  Operator=tan
  Trigonometric Function3 : Trigonometry  Operator=cos
  psi0 : Constant  Value=psi0
  psi : Outport
  wires:
  Integrator/1 -> psi/1, Trigonometric Function3/1, Trigonometric Function/1
  Product/1 -> Sum/1
  phi/1 -> Trigonometric Function2/1
  Trigonometric Function2/1 -> Product/2
  wq3/1 -> Product1/2
  Trigonometric Function3/1 -> Product1/1
  Product1/1 -> Add/1
  Add/1 -> Product/1
  Trigonometric Function/1 -> Product2/1
  wq2/1 -> Product2/2
  Product2/1 -> Add/2
  wq1/1 -> Sum/2
  Sum/1 -> Integrator/1
  psi0/1 -> Integrator/2

== system lazo_cerrado_cir/Subsystem1/Cinemática/Ángulos De Euler/Subsystem2 ==
  psi : Inport
  wq2 : Inport  Port=2
  wq3 : Inport  Port=3
  Integrator : DiscreteIntegrator  InitialConditionSource=external  SampleTime=Ts  ICPrevOutput=DiscIntNeverNeededParam  ICPrevScaledInput=DiscIntNeverNeededParam  mask(DiscretizedDiscreteIntegrator){}
      mask init:
      | %zoh
  Product : Product  RndMeth=Zero
  Product1 : Product  RndMeth=Zero
  Subtract : Sum  Inputs=+-
  Trigonometric Function : Trigonometry  Operator=cos
  Trigonometric Function1 : Trigonometry
  phi0 : Constant  Value=phi0
  phi : Outport
  wires:
  Integrator/1 -> phi/1
  Subtract/1 -> Integrator/1
  Product/1 -> Subtract/1
  Product1/1 -> Subtract/2
  Trigonometric Function/1 -> Product/1
  psi/1 -> Trigonometric Function/1, Trigonometric Function1/1
  Trigonometric Function1/1 -> Product1/1
  wq2/1 -> Product/2
  wq3/1 -> Product1/2
  phi0/1 -> Integrator/2

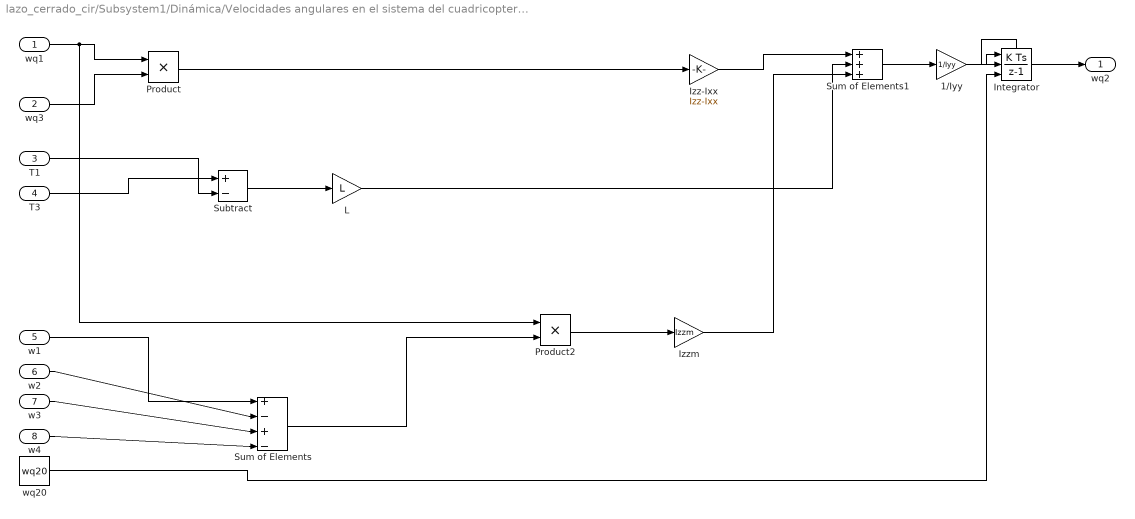
== system lazo_cerrado_cir/Subsystem1/Dinámica/Velocidades angulares en el sistema del cuadricoptero/Subsystem10 ==
  wq1 : Inport
  wq3 : Inport  Port=2
  T1 : Inport  Port=3
  T3 : Inport  Port=4
  w1 : Inport  Port=5
  w2 : Inport  Port=6
  w3 : Inport  Port=7
  w4 : Inport  Port=8
  1/Iyy : Gain  Gain=1/Iyy
  Integrator : DiscreteIntegrator  ExternalReset=either  InitialConditionSource=external  SampleTime=Ts  ShowStatePort=on  ICPrevOutput=DiscIntNeverNeededParam  ICPrevScaledInput=DiscIntNeverNeededParam  mask(DiscretizedDiscreteIntegrator){}
      mask init:
      | %zoh
  Izz-Ixx : Gain  Gain=Izz-Ixx
  Izzm : Gain  Gain=Izzm
  L : Gain  Gain=L
  Product : Product  RndMeth=Zero
  Product2 : Product  RndMeth=Zero
  Subtract : Sum  Inputs=+-
  Sum of Elements : Sum  Inputs=+|-|+|-|
  Sum of Elements1 : Sum  Inputs=3
  wq20 : Constant  Value=wq20
  wq2 : Outport
  wires:
  wq1/1 -> Product/1, Product2/1
  wq3/1 -> Product/2
  Product/1 -> Izz-Ixx/1
  T3/1 -> Subtract/1
  T1/1 -> Subtract/2
  w1/1 -> Sum of Elements/1
  w2/1 -> Sum of Elements/2
  w3/1 -> Sum of Elements/3
  w4/1 -> Sum of Elements/4
  Sum of Elements/1 -> Product2/2
  Product2/1 -> Izzm/1
  Izzm/1 -> Sum of Elements1/3
  Sum of Elements1/1 -> 1/Iyy/1
  1/Iyy/1 -> Integrator/1
  Integrator/1 -> wq2/1
  Subtract/1 -> L/1
  Izz-Ixx/1 -> Sum of Elements1/1
  L/1 -> Sum of Elements1/2
  wq20/1 -> Integrator/3
  Integrator/State -> Integrator/2

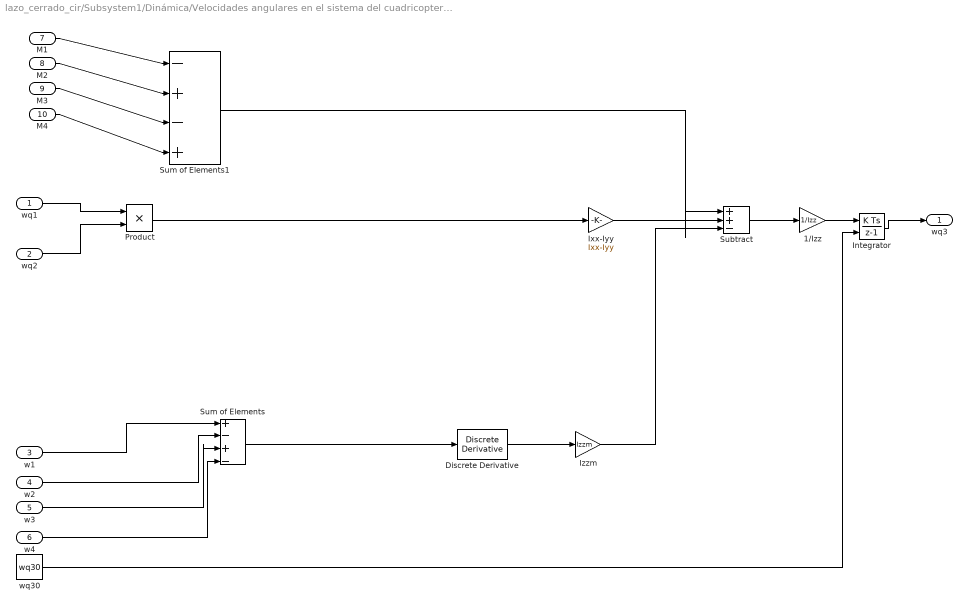
== system lazo_cerrado_cir/Subsystem1/Dinámica/Velocidades angulares en el sistema del cuadricoptero/Subsystem11 ==
  wq1 : Inport
  wq2 : Inport  Port=2
  w1 : Inport  Port=3
  w2 : Inport  Port=4
  w3 : Inport  Port=5
  w4 : Inport  Port=6
  M1 : Inport  Port=7
  M2 : Inport  Port=8
  M3 : Inport  Port=9
  M4 : Inport  Port=10
  1/Izz : Gain  Gain=1/Izz
  Discrete Derivative : simulink/Discrete/Discrete Derivative  SystemSampleTime=-1  gainval=1.0  ICPrevScaledInput=0.0  OutMin=[]  OutMax=[]  OutDataType=fixdt(1, 16)  OutScaling=2^-10  DoSatur=off
  Integrator : DiscreteIntegrator  InitialConditionSource=external  SampleTime=Ts  ICPrevOutput=DiscIntNeverNeededParam  ICPrevScaledInput=DiscIntNeverNeededParam  mask(DiscretizedDiscreteIntegrator){}
      mask init:
      | %zoh
  Ixx-Iyy : Gain  Gain=Ixx-Iyy
  Izzm : Gain  Gain=Izzm
  Product : Product  RndMeth=Zero
  Subtract : Sum  Inputs=++-
  Sum of Elements : Sum  Inputs=+|-|+|-|
  Sum of Elements1 : Sum  Inputs=-|+|-|+|
  wq30 : Constant  Value=wq30
  wq3 : Outport
  wires:
  wq1/1 -> Product/1
  wq2/1 -> Product/2
  Product/1 -> Ixx-Iyy/1
  w4/1 -> Sum of Elements/4
  Subtract/1 -> 1/Izz/1
  1/Izz/1 -> Integrator/1
  Integrator/1 -> wq3/1
  wq30/1 -> Integrator/2
  w1/1 -> Sum of Elements/1
  w2/1 -> Sum of Elements/2
  w3/1 -> Sum of Elements/3
  Sum of Elements/1 -> Discrete Derivative/1
  M1/1 -> Sum of Elements1/1
  M2/1 -> Sum of Elements1/2
  M3/1 -> Sum of Elements1/3
  M4/1 -> Sum of Elements1/4
  Sum of Elements1/1 -> Subtract/1
  Izzm/1 -> Subtract/3
  Ixx-Iyy/1 -> Subtract/2
  Discrete Derivative/1 -> Izzm/1

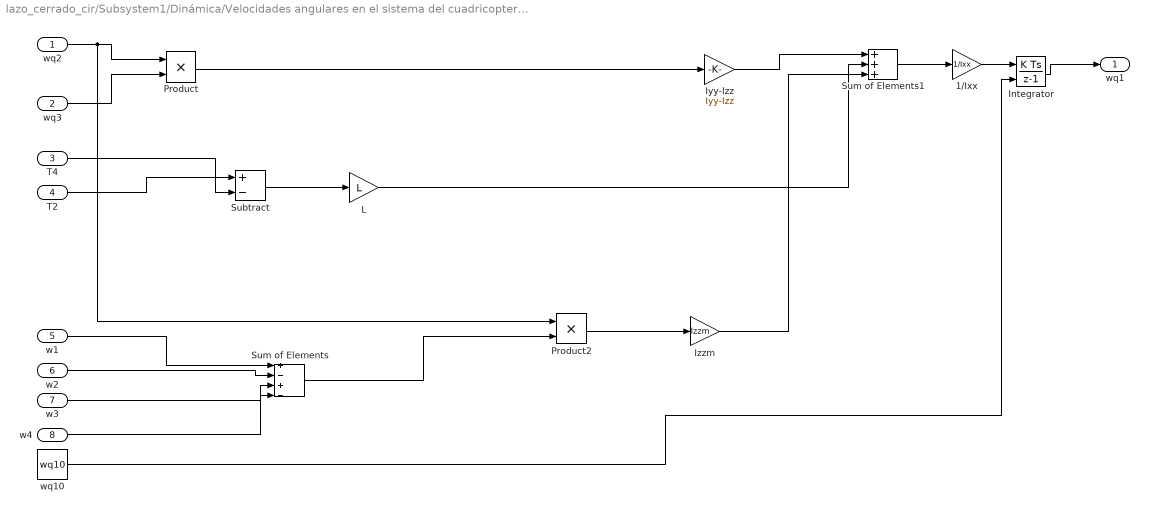
== system lazo_cerrado_cir/Subsystem1/Dinámica/Velocidades angulares en el sistema del cuadricoptero/Subsystem9 ==
  wq2 : Inport
  wq3 : Inport  Port=2
  T4 : Inport  Port=3
  T2 : Inport  Port=4
  w1 : Inport  Port=5
  w2 : Inport  Port=6
  w3 : Inport  Port=7
  w4 : Inport  Port=8
  1/Ixx : Gain  Gain=1/Ixx
  Integrator : DiscreteIntegrator  InitialConditionSource=external  SampleTime=Ts  ICPrevOutput=DiscIntNeverNeededParam  ICPrevScaledInput=DiscIntNeverNeededParam  mask(DiscretizedDiscreteIntegrator){}
      mask init:
      | %zoh
  Iyy-Izz : Gain  Gain=Iyy-Izz
  Izzm : Gain  Gain=Izzm
  L : Gain  Gain=L
  Product : Product  RndMeth=Zero
  Product2 : Product  RndMeth=Zero
  Subtract : Sum  Inputs=+-
  Sum of Elements : Sum  Inputs=+|-|+|-
  Sum of Elements1 : Sum  Inputs=3
  wq10 : Constant  Value=wq10
  wq1 : Outport
  wires:
  wq2/1 -> Product/1, Product2/1
  wq3/1 -> Product/2
  Product/1 -> Iyy-Izz/1
  T2/1 -> Subtract/1
  T4/1 -> Subtract/2
  w1/1 -> Sum of Elements/1
  w3/1 -> Sum of Elements/3
  w4/1 -> Sum of Elements/4
  Sum of Elements/1 -> Product2/2
  Product2/1 -> Izzm/1
  Izzm/1 -> Sum of Elements1/3
  Sum of Elements1/1 -> 1/Ixx/1
  1/Ixx/1 -> Integrator/1
  Integrator/1 -> wq1/1
  Subtract/1 -> L/1
  Iyy-Izz/1 -> Sum of Elements1/1
  L/1 -> Sum of Elements1/2
  w2/1 -> Sum of Elements/2
  wq10/1 -> Integrator/2

== system lazo_cerrado_cir/Subsystem1/Dinámica/Velocidades en el sistema del cuadricóptero/Subsystem6 ==
  phi : Inport
  wq2 : Inport  Port=2
  wq3 : Inport  Port=3
  vq2 : Inport  Port=4
  vq3 : Inport  Port=5
  Add : Sum
  Integrator : DiscreteIntegrator  InitialConditionSource=external  SampleTime=Ts  ICPrevOutput=DiscIntNeverNeededParam  ICPrevScaledInput=DiscIntNeverNeededParam  mask(DiscretizedDiscreteIntegrator){}
      mask init:
      | %zoh
  Product : Product  RndMeth=Zero
  Product1 : Product  RndMeth=Zero
  Subtract : Sum  Inputs=+-
  Trigonometric Function4 : Trigonometry
  gravedad : Gain  Gain=g
  vq10 : Constant  Value=vq10
  vq1 : Outport
  wires:
  phi/1 -> Trigonometric Function4/1
  vq2/1 -> Product/2
  wq3/1 -> Product/1
  vq3/1 -> Product1/2
  wq2/1 -> Product1/1
  Product/1 -> Subtract/1
  Product1/1 -> Subtract/2
  Trigonometric Function4/1 -> gravedad/1
  gravedad/1 -> Add/1
  Subtract/1 -> Add/2
  Add/1 -> Integrator/1
  Integrator/1 -> vq1/1
  vq10/1 -> Integrator/2

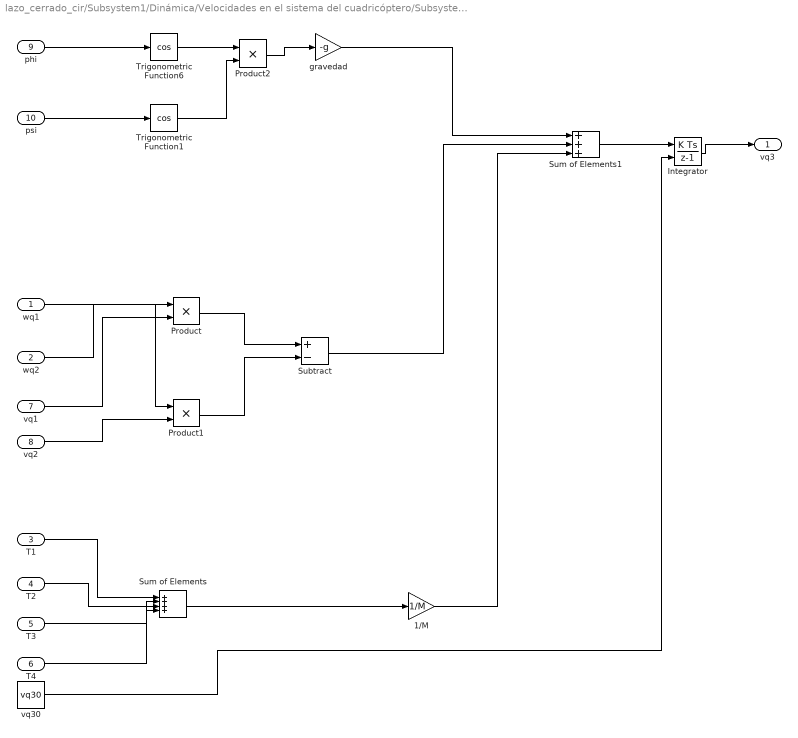
== system lazo_cerrado_cir/Subsystem1/Dinámica/Velocidades en el sistema del cuadricóptero/Subsystem7 ==
  wq1 : Inport
  wq2 : Inport  Port=2
  T1 : Inport  Port=3
  T2 : Inport  Port=4
  T3 : Inport  Port=5
  T4 : Inport  Port=6
  vq1 : Inport  Port=7
  vq2 : Inport  Port=8
  phi : Inport  Port=9
  psi : Inport  Port=10
  1/M : Gain  Gain=1/M
  Integrator : DiscreteIntegrator  InitialConditionSource=external  SampleTime=Ts  ICPrevOutput=DiscIntNeverNeededParam  ICPrevScaledInput=DiscIntNeverNeededParam  mask(DiscretizedDiscreteIntegrator){}
      mask init:
      | %zoh
  Product : Product  RndMeth=Zero
  Product1 : Product  RndMeth=Zero
  Product2 : Product  RndMeth=Zero
  Subtract : Sum  Inputs=+-
  Sum of Elements : Sum  Inputs=4
  Sum of Elements1 : Sum  Inputs=3
  Trigonometric Function1 : Trigonometry  Operator=cos
  Trigonometric Function6 : Trigonometry  Operator=cos
  gravedad : Gain  Gain=-g
  vq30 : Constant  Value=vq30
  vq3 : Outport
  wires:
  T1/1 -> Sum of Elements/1
  T2/1 -> Sum of Elements/2
  T3/1 -> Sum of Elements/3
  T4/1 -> Sum of Elements/4
  Sum of Elements/1 -> 1/M/1
  vq1/1 -> Product/2
  wq2/1 -> Product/1
  vq2/1 -> Product1/2
  wq1/1 -> Product1/1
  Product/1 -> Subtract/1
  Product1/1 -> Subtract/2
  phi/1 -> Trigonometric Function6/1
  psi/1 -> Trigonometric Function1/1
  Trigonometric Function1/1 -> Product2/2
  gravedad/1 -> Sum of Elements1/1
  Subtract/1 -> Sum of Elements1/2
  1/M/1 -> Sum of Elements1/3
  Sum of Elements1/1 -> Integrator/1
  Integrator/1 -> vq3/1
  Trigonometric Function6/1 -> Product2/1
  Product2/1 -> gravedad/1
  vq30/1 -> Integrator/2

== system lazo_cerrado_cir/Subsystem1/Dinámica/Velocidades en el sistema del cuadricóptero/Subsystem8 ==
  phi : Inport
  wq3 : Inport  Port=2
  wq1 : Inport  Port=3
  vq3 : Inport  Port=4
  vq1 : Inport  Port=5
  psi : Inport  Port=6
  Add : Sum
  Integrator : DiscreteIntegrator  InitialConditionSource=external  SampleTime=Ts  ICPrevOutput=DiscIntNeverNeededParam  ICPrevScaledInput=DiscIntNeverNeededParam  mask(DiscretizedDiscreteIntegrator){}
      mask init:
      | %zoh
  Product : Product  RndMeth=Zero
  Product1 : Product  RndMeth=Zero
  Product2 : Product  RndMeth=Zero
  Subtract : Sum  Inputs=+-
  Trigonometric Function1 : Trigonometry
  Trigonometric Function4 : Trigonometry  Operator=cos
  gravedad : Gain  Gain=-g
  vq20 : Constant  Value=vq20
  vq2 : Outport
  wires:
  phi/1 -> Trigonometric Function4/1
  vq3/1 -> Product/2
  wq1/1 -> Product/1
  vq1/1 -> Product1/2
  wq3/1 -> Product1/1
  Product/1 -> Subtract/1
  Product1/1 -> Subtract/2
  gravedad/1 -> Add/1
  Subtract/1 -> Add/2
  Add/1 -> Integrator/1
  Integrator/1 -> vq2/1
  psi/1 -> Trigonometric Function1/1
  Trigonometric Function1/1 -> Product2/2
  Trigonometric Function4/1 -> Product2/1
  Product2/1 -> gravedad/1
  vq20/1 -> Integrator/2
